simulink model "TESTS"  (R2022b)
settings: Solver=ode4  StartTime=0.0  StopTime=10.0  FixedStep=1e-4  RelTol=1e-3
values from neighbouring files (symbols this model uses):
  cel_serie = 6    [init_VE_EPRM_24_25.m]
  ke = 0.107    [init_VE_EPRM_24_25.m]
  ki = ke    (= 0.107)    [init_VE_EPRM_24_25.m]
  Kie = Kpe/taue    (= 9.6)    [init_VE_EPRM_24_25.m]
  Kpe = taue/(gaine*tftbe)    (= 0.045)    [init_VE_EPRM_24_25.m]
  Kpm = Mv/taum    (= 8850)    [init_VE_EPRM_24_25.m]
  kred = 75/22    (= 3.40909090909)    [init_VE_EPRM_24_25.m]
  Lmcc = vbat/(2*fdec*Deltai)    (= 0.00015)    [init_VE_EPRM_24_25.m]
  mod_serie = 4    [init_VE_EPRM_24_25.m]
  Mv = 295    [init_VE_EPRM_24_25.m]
  n = 0.92    [init_VE_EPRM_24_25.m]
  r = (279.4*10^-3)/2    (= 0.1397)    [init_VE_EPRM_24_25.m]
  Rcell = 0.53*10^-3    (= 0.00053)    [init_VE_EPRM_24_25.m]
  Rmcc = 0.032    [init_VE_EPRM_24_25.m]
  Voc = 2    [init_VE_EPRM_24_25.m]
libraries: slpidlib x1, simulink x1
settings Model: Creator=ZinouAb  LastModifiedBy=ZinouAb

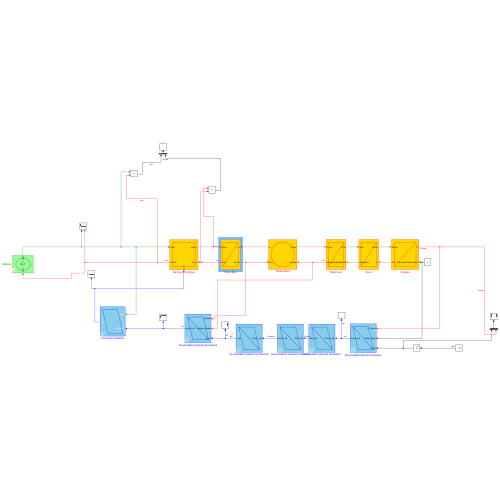
[thumbnail: Simulink's stored preview of the top-level diagram]
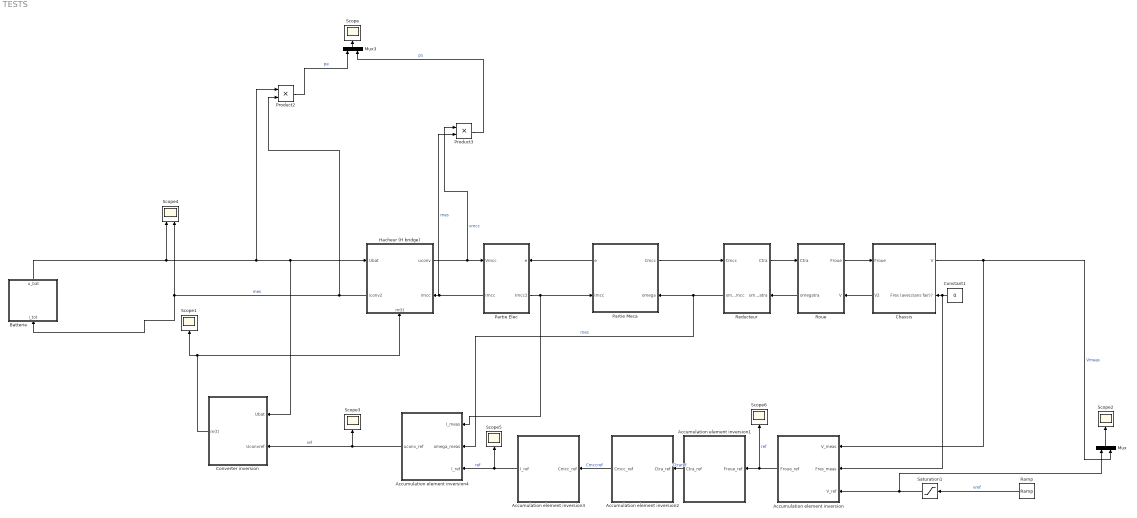
== system TESTS ==
  Accumulation element inversion : Subsystem  AncestorBlock=simulink/SMC/Asservissement Correcteur IP
      settings: LibrarySourceBlock=|
      | simulink/SMC/Asservissement
      | Correcteur IP
      mask Display: plot(0,0,100,100, [10,30,90,70,10,90],[90,10,10,90,90,10])
  Accumulation element inversion1 : Subsystem  AncestorBlock=simulink/SMC/Asservissement Correcteur IP
      settings: LibrarySourceBlock=|
      | simulink/SMC/Asservissement
      | Correcteur IP
      mask Display: plot(0,0,100,100, [10,30,90,70,10,90],[90,10,10,90,90,10])
  Accumulation element inversion2 : Subsystem  AncestorBlock=simulink/SMC/Asservissement Correcteur IP
      settings: LibrarySourceBlock=|
      | simulink/SMC/Asservissement
      | Correcteur IP
      mask Display: plot(0,0,100,100, [10,30,90,70,10,90],[90,10,10,90,90,10])
  Accumulation element inversion3 : Subsystem  AncestorBlock=simulink/SMC/Asservissement Correcteur IP
      settings: LibrarySourceBlock=|
      | simulink/SMC/Asservissement
      | Correcteur IP
      mask Display: plot(0,0,100,100, [10,30,90,70,10,90],[90,10,10,90,90,10])
  Accumulation element inversion4 : Subsystem  AncestorBlock=simulink/SMC/Asservissement Correcteur IP
      settings: LibrarySourceBlock=|
      | simulink/SMC/Asservissement
      | Correcteur IP
      mask Display: plot(0,0,100,100, [10,30,90,70,10,90],[90,10,10,90,90,10])
  Batterie : Subsystem  AncestorBlock=simulink/REM/SE
      settings: LibrarySourceBlock=simulink/REM/SE
      mask Display:
      | plot(0,0,100,100, 1.2*[50,57.68,60.77,63.08,64.97,66.58,68,69.26,70.4, 	71.42,72.36,78.28,80,78.28,72.36,71.42,70.4, 	69.26,68,66.58,64.97,63.08,60.77,57.68,50,42.32, 	39.23,36.92,35.03,33.42,32,30.74,29.6,28.58, 	27.64,21.72,20,21.72,27.64,28.58,29.6,30.74,32, 	33.42,35.03,36.92,39.23,42.32,50]-10, 1.2*[20,21,22,23,24,25,26,27,28,29,30,40,50,60,70,71,72, 	73,74,75,76,77,78,79,80,79,78,77,76,75,74,73,72, 	71,70,60,50,40,30,29,28,27,26,25,24,23,22,21,20]-10)
      | disp('BAT')
  Chassis : Subsystem
      settings: PortSchema="{\"entries\":[{\"content\":{\"sides\":[{\"content\":{\"connectorIds\":[\"In1\",\"Out2\"]},\"type\":\"ConnectorPlacement.EquallySpacedRectSide\",\"uuid\":\"2a4fefbc-7af2-45ac-94e1-720f9d1a181b\"},{\"content\":{\"connectorIds\":[\"Out1\",\"In2\"],\"side\":\"RIGHT\"},\"type\":\"ConnectorPlacement.EquallySpacedRectSide\",\"uuid\":\"47213f8a-38f1-43b2-8885-5842ee71090a\"},{\"content\":{\"connectorIds\":[],\"side\":\"TOP\"},\"type\":\"ConnectorPlacement.EquallySpacedRectSide\",\"uuid\":\"9ff55915-a798-409c-870e-d15a860382f9\"}]},\"type\":\"ConnectorPlacement.EquallySpacedConnector\",\"uuid\":\"647a32d4-94be-4190-bdc8-90a1a32d4cbf\"}],\"packageUris\":[\"http://schema.mathworks.com/mf0/Connector/R2020b\"],\"version\":\"1.0\"}"
      mask Display: plot(0,0,100,100,[10,10,90,90,10],[90,10,10,90,90], [10,90],[10,90])
  Constant1 : Constant  Value=0
  Converter inversion : Subsystem  AncestorBlock=simulink/SMC/Inversion EC avec mesure
      settings: LibrarySourceBlock=|
      | simulink/SMC/Inversion EC
      | avec mesure
      mask Display: plot(0,0,100,100,[10,30,90,70,10],[90,10,10,90,90])
  Hacheur (H bridge) : Subsystem
      settings: PortSchema="{\"entries\":[{\"content\":{\"sides\":[{\"content\":{\"connectorIds\":[\"In1\",\"Out2\"]},\"type\":\"ConnectorPlacement.EquallySpacedRectSide\",\"uuid\":\"15c37a82-4fae-4dd0-ab5a-78fb718c05e2\"},{\"content\":{\"connectorIds\":[\"Out1\",\"In3\"],\"side\":\"RIGHT\"},\"type\":\"ConnectorPlacement.EquallySpacedRectSide\",\"uuid\":\"2898708c-5198-4fba-9c94-abd5bb9e9c70\"},{\"content\":{\"connectorIds\":[],\"side\":\"TOP\"},\"type\":\"ConnectorPlacement.EquallySpacedRectSide\",\"uuid\":\"a769b592-c34b-45c3-8b04-17631095b399\"},{\"content\":{\"connectorIds\":[\"In2\"],\"side\":\"BOTTOM\"},\"type\":\"ConnectorPlacement.EquallySpacedRectSide\",\"uuid\":\"3f87bc4b-31a4-497c-9119-c9de1168f7cf\"}]},\"type\":\"ConnectorPlacement.EquallySpacedConnector\",\"uuid\":\"cf4da0bd-1e1f-410f-93a1-c54772eba95e\"}],\"packageUris\":[\"http://schema.mathworks.com/mf0/Connector/R2020b\"],\"version\":\"1.0\"}"
      mask Display: plot(0,0,100,100,[10,10,90,90,10],[90,10,10,90,90])
  Mux : Mux  Inputs=2
  Mux3 : Mux  Inputs=2
  Partie Elec : Subsystem
      settings: PortSchema="{\"entries\":[{\"content\":{\"sides\":[{\"content\":{\"connectorIds\":[\"In1\",\"Out2\"]},\"type\":\"ConnectorPlacement.EquallySpacedRectSide\",\"uuid\":\"2a4fefbc-7af2-45ac-94e1-720f9d1a181b\"},{\"content\":{\"connectorIds\":[\"In2\",\"Out1\"],\"side\":\"RIGHT\"},\"type\":\"ConnectorPlacement.EquallySpacedRectSide\",\"uuid\":\"47213f8a-38f1-43b2-8885-5842ee71090a\"},{\"content\":{\"connectorIds\":[],\"side\":\"TOP\"},\"type\":\"ConnectorPlacement.EquallySpacedRectSide\",\"uuid\":\"9ff55915-a798-409c-870e-d15a860382f9\"}]},\"type\":\"ConnectorPlacement.EquallySpacedConnector\",\"uuid\":\"647a32d4-94be-4190-bdc8-90a1a32d4cbf\"}],\"packageUris\":[\"http://schema.mathworks.com/mf0/Connector/R2020b\"],\"version\":\"1.0\"}"
      mask Display: plot(0,0,100,100,[10,10,90,90,10],[90,10,10,90,90], [10,90],[10,90])
  Partie Meca : Subsystem
      settings: PortSchema="{\"entries\":[{\"content\":{\"sides\":[{\"content\":{\"connectorIds\":[\"Out2\",\"In1\"]},\"type\":\"ConnectorPlacement.EquallySpacedRectSide\",\"uuid\":\"2a4fefbc-7af2-45ac-94e1-720f9d1a181b\"},{\"content\":{\"connectorIds\":[\"Out1\",\"In2\"],\"side\":\"RIGHT\"},\"type\":\"ConnectorPlacement.EquallySpacedRectSide\",\"uuid\":\"47213f8a-38f1-43b2-8885-5842ee71090a\"},{\"content\":{\"connectorIds\":[],\"side\":\"TOP\"},\"type\":\"ConnectorPlacement.EquallySpacedRectSide\",\"uuid\":\"9ff55915-a798-409c-870e-d15a860382f9\"}]},\"type\":\"ConnectorPlacement.EquallySpacedConnector\",\"uuid\":\"647a32d4-94be-4190-bdc8-90a1a32d4cbf\"}],\"packageUris\":[\"http://schema.mathworks.com/mf0/Connector/R2020b\"],\"version\":\"1.0\"}"
      mask Display: plot(0,0,100,100, 1.4*[50,57.68,60.77,63.08,64.97,66.58,68,69.26,70.4, 	71.42,72.36,78.28,80,78.28,72.36,71.42,70.4, 	69.26,68,66.58,64.97,63.08,60.77,57.68,50,42.32, 	39.23,36.92,35.03,33.42,32,30.74,29.6,28.58, 	27.64,21.72,20,21.72,27.64,28.58,29.6,30.74,32, 	33.42,35.03,36.92,39.23,42.32,50]-20, 1.4*[20,21,22,23,24,25,26,27,28,29,30,40,50,60,70,71,72, 	73,74,75,76,77,78,79,80,79,78,77,76,75,74,73,72, 	71,70,60,50,40,30,29,28,27,26,25,24,23,22,21,20]-20)
  Product2 : Product
  Product3 : Product
  Ramp : simulink/Sources/Ramp  slope=1  start=1  InitialOutput=0
  Reducteur : Subsystem
      settings: PortSchema="{\"entries\":[{\"content\":{\"sides\":[{\"content\":{\"connectorIds\":[\"In1\",\"Out2\"]},\"type\":\"ConnectorPlacement.EquallySpacedRectSide\",\"uuid\":\"2a4fefbc-7af2-45ac-94e1-720f9d1a181b\"},{\"content\":{\"connectorIds\":[\"Out1\",\"In2\"],\"side\":\"RIGHT\"},\"type\":\"ConnectorPlacement.EquallySpacedRectSide\",\"uuid\":\"47213f8a-38f1-43b2-8885-5842ee71090a\"},{\"content\":{\"connectorIds\":[],\"side\":\"TOP\"},\"type\":\"ConnectorPlacement.EquallySpacedRectSide\",\"uuid\":\"9ff55915-a798-409c-870e-d15a860382f9\"}]},\"type\":\"ConnectorPlacement.EquallySpacedConnector\",\"uuid\":\"647a32d4-94be-4190-bdc8-90a1a32d4cbf\"}],\"packageUris\":[\"http://schema.mathworks.com/mf0/Connector/R2020b\"],\"version\":\"1.0\"}"
      mask Display: plot(0,0,100,100,[10,10,90,90,10],[90,10,10,90,90], [10,90],[10,90])
  Roue : Subsystem
      settings: PortSchema="{\"entries\":[{\"content\":{\"sides\":[{\"content\":{\"connectorIds\":[\"In1\",\"Out2\"]},\"type\":\"ConnectorPlacement.EquallySpacedRectSide\",\"uuid\":\"2a4fefbc-7af2-45ac-94e1-720f9d1a181b\"},{\"content\":{\"connectorIds\":[\"Out1\",\"In2\"],\"side\":\"RIGHT\"},\"type\":\"ConnectorPlacement.EquallySpacedRectSide\",\"uuid\":\"47213f8a-38f1-43b2-8885-5842ee71090a\"},{\"content\":{\"connectorIds\":[],\"side\":\"TOP\"},\"type\":\"ConnectorPlacement.EquallySpacedRectSide\",\"uuid\":\"9ff55915-a798-409c-870e-d15a860382f9\"}]},\"type\":\"ConnectorPlacement.EquallySpacedConnector\",\"uuid\":\"647a32d4-94be-4190-bdc8-90a1a32d4cbf\"}],\"packageUris\":[\"http://schema.mathworks.com/mf0/Connector/R2020b\"],\"version\":\"1.0\"}"
      mask Display: plot(0,0,100,100,[10,10,90,90,10],[90,10,10,90,90], [10,90],[10,90])
  Saturation1 : Saturate  UpperLimit=1  LowerLimit=-1  LinearizeAsGain=off
  Scope{,1..3,5..6} (6 alike) : Scope
  Scope4 : Scope  NumInputPorts=2
  wires:
  Accumulation element inversion4/1(uconv_ref) -> Scope3/1, Converter inversion/2("Uconvref ")  "ref"
  Converter inversion/1(m(t)) -> Hacheur (H bridge)/2(m(t)), Scope1/1
  Partie Elec/1(Imcc2) -> Partie Meca/1(Imcc), Accumulation element inversion4/1(I_meas)
  Product3/1 -> Mux3/2  "ps"
  Mux3/1 -> Scope/1
  Product2/1 -> Mux3/1  "pe"
  Hacheur (H bridge)/1("uconv ") -> Product3/1, Partie Elec/1(Vmcc)  "vmcc"
  Mux/1 -> Scope2/1
  Partie Meca/2(e) -> Partie Elec/2(e)
  Reducteur/1(Ctra) -> Roue/1(Ctra)
  Roue/2(omegatra) -> Reducteur/2(omegatra)
  Roue/1(Froue) -> Chassis/1(Froue)
  Chassis/2(V2) -> Roue/2(V)
  Partie Meca/1(Cmcc) -> Reducteur/1(Cmcc)
  Reducteur/2(omegamcc) -> Accumulation element inversion4/2(omega_meas), Partie Meca/2(omega)  "mes"
  Constant1/1 -> Accumulation element inversion/2(Fres_meas), Chassis/2(Fres (avec/sans fair)?)
  Chassis/1(V) -> Mux/2, Accumulation element inversion/1(V_meas)  "Vmeas"
  Accumulation element inversion1/1(Ctra_ref) -> Accumulation element inversion2/1(Ctra_ref)  "Ctraref"
  Accumulation element inversion2/1(Cmcc_ref) -> Accumulation element inversion3/1(Cmcc_ref)  "Cmccref"
  Hacheur (H bridge)/2(iconv2) -> Product2/2, Batterie/1(i_tot), Scope4/2  "mes"
  Batterie/1(u_bat) -> Scope4/1, Product2/1, Converter inversion/1(Ubat), Hacheur (H bridge)/1("Ubat ")
  Partie Elec/2(Imcc) -> Hacheur (H bridge)/3("imcc "), Product3/2  "mes"
  Accumulation element inversion3/1(I_ref) -> Scope5/1, Accumulation element inversion4/3(I_ref)  "ref"
  Accumulation element inversion/1(Froue_ref) -> Scope6/1, Accumulation element inversion1/1(Froue_ref)  "ref"
  Saturation1/1 -> Mux/1, Accumulation element inversion/3(V_ref)
  Ramp/1 -> Saturation1/1  "vref"

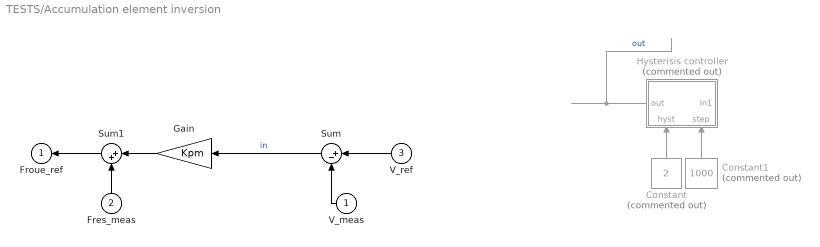
== system TESTS/Accumulation element inversion ==
  V_meas : Inport
  Fres_meas : Inport  Port=2
  V_ref : Inport  Port=3
  Constant : Constant  Commented=on  Value=2
  Constant1 : Constant  Commented=on  Value=1000
  Gain : Gain  Gain=Kpm
  Hysterisis controller : Subsystem  Commented=on
      settings: PortSchema="{\"entries\":[{\"content\":{\"sides\":[{\"content\":{\"connectorIds\":[\"In1\"]},\"type\":\"ConnectorPlacement.EquallySpacedRectSide\",\"uuid\":\"f66aa083-2ee8-4426-b441-0f8ce3c91bc6\"},{\"content\":{\"connectorIds\":[\"Out1\"],\"side\":\"RIGHT\"},\"type\":\"ConnectorPlacement.EquallySpacedRectSide\",\"uuid\":\"e535ff9d-11f2-429a-8d26-bff265e6dce4\"},{\"content\":{\"connectorIds\":[\"In2\",\"In3\"],\"side\":\"TOP\"},\"type\":\"ConnectorPlacement.EquallySpacedRectSide\",\"uuid\":\"3bf3f486-5ffc-4655-8aef-50265858aab1\"},{\"content\":{\"connectorIds\":[],\"side\":\"BOTTOM\"},\"type\":\"ConnectorPlacement.EquallySpacedRectSide\",\"uuid\":\"619b2421-7bbc-4c41-b693-a17d0c478cc9\"}]},\"type\":\"ConnectorPlacement.EquallySpacedConnector\",\"uuid\":\"4c23f3cf-154a-4c58-b671-46cc18db332d\"}],\"packageUris\":[\"http://schema.mathworks.com/mf0/Connector/R2020b\"],\"version\":\"1.0\"}"
  Sum : Sum  Inputs=|+-
  Sum1 : Sum  Inputs=|++
  Froue_ref : Outport  InitialOutput=0
  wires:
  Hysterisis controller/1(out) -> ?  "out"
  Sum/1 -> Gain/1  "in"
  Constant/1 -> Hysterisis controller/3(hyst)
  Fres_meas/1 -> Sum1/2
  Sum1/1 -> Froue_ref/1
  ? -> Hysterisis controller/1(In1)  "in"
  Constant1/1 -> Hysterisis controller/2(step)
  V_ref/1 -> Sum/1
  V_meas/1 -> Sum/2
  Gain/1 -> Sum1/1

== system TESTS/Accumulation element inversion1 ==
  Froue_ref : Inport
  Gain : Gain  Gain=r
  Ctra_ref : Outport  InitialOutput=0
  wires:
  Gain/1 -> Ctra_ref/1
  Froue_ref/1 -> Gain/1

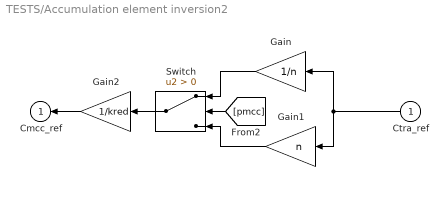
== system TESTS/Accumulation element inversion2 ==
  Ctra_ref : Inport
  Gain : Gain  Gain=1/n
  Gain1 : Gain  Gain=n
  Gain2 : Gain  Gain=1/kred
  Switch : Switch  Criteria=u2 > Threshold  SaturateOnIntegerOverflow=off  InputSameDT=off
  Cmcc_ref : Outport  InitialOutput=0
  wires:
  Switch/1 -> Gain2/1
  Ctra_ref/1 -> Gain/1, Gain1/1
  [pmcc] -> Switch/2
  Gain/1 -> Switch/1
  Gain1/1 -> Switch/3
  Gain2/1 -> Cmcc_ref/1

== system TESTS/Accumulation element inversion3 ==
  Cmcc_ref : Inport
  Gain : Gain  Gain=1/ki
  I_ref : Outport  InitialOutput=0
  wires:
  Gain/1 -> I_ref/1
  Cmcc_ref/1 -> Gain/1

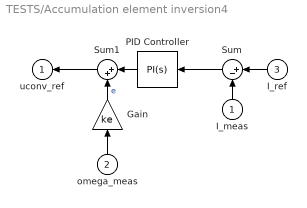
== system TESTS/Accumulation element inversion4 ==
  I_meas : Inport
  omega_meas : Inport  Port=2
  I_ref : Inport  Port=3
  Gain : Gain  Gain=ke
  PID Controller : slpidlib/PID Controller  Controller=PI  Form=Parallel  TimeDomain=Continuous-time  UseExternalTs=off  SampleTime=-1  IntegratorMethod=Forward Euler  FilterMethod=Forward Euler  ControllerParametersSource=internal  P=Kpe  I=Kie  UseKiTs=off  D=0  N=100  UseFilter=on  TunerSelectOption=Transfer Function Based (PID Tuner App)  InitialConditionSource=internal  InitialConditionForIntegrator=0  InitialConditionForFilter=0  DifferentiatorICPrevScaledInput=0  ExternalReset=none  TrackingMode=off  Kt=1  LimitOutput=off  SatLimitsSource=internal  UpperSaturationLimit=inf  LowerSaturationLimit=-inf  LinearizeAsGain=on  AntiWindupMode=none  Kb=1  LimitIntegrator=off  UpperIntegratorSaturationLimit=inf  LowerIntegratorSaturationLimit=-inf  POutMin=[]  POutMax=[]  IOutMin=[]  IOutMax=[]  DOutMin=[]  DOutMax=[]  NOutMin=[]  NOutMax=[]  SumOutMin=[]  SumOutMax=[]  SaturationOutMin=[]  SaturationOutMax=[]  PParamMin=[]  PParamMax=[]  IParamMin=[]  IParamMax=[]  DParamMin=[]  DParamMax=[]  NParamMin=[]  NParamMax=[]  KbParamMin=[]  KbParamMax=[]  KtParamMin=[]  KtParamMax=[]  KbOutMin=[]  KbOutMax=[]  KtOutMin=[]  KtOutMax=[]  IntegratorOutMin=[]  IntegratorOutMax=[]  FilterOutMin=[]  FilterOutMax=[]  SumI1OutMin=[]  SumI1OutMax=[]  SumI2OutMin=[]  SumI2OutMax=[]  SumI3OutMin=[]  SumI3OutMax=[]  SumI4OutMin=[]  SumI4OutMax=[]  SumDOutMin=[]  SumDOutMax=[]  DifferentiatorOutMin=[]  DifferentiatorOutMax=[]  FilterDiffOutCoefMin=[]  FilterDiffOutCoefMax=[]  ReciprocalOutMin=[]  ReciprocalOutMax=[]  SumDenOutMin=[]  SumDenOutMax=[]  SumNumOutMin=[]  SumNumOutMax=[]  DivideOutMin=[]  DivideOutMax=[]  UdiffTsProdOutMin=[]  UdiffTsProdOutMax=[]  NTsProdOutMin=[]  NTsProdOutMax=[]  UintegralTsProdOutMin=[]  UintegralTsProdOutMax=[]  UngainTsProdOutMin=[]  UngainTsProdOutMax=[]  ClampingZeroOutDataTypeStr=Inherit: Inherit via back propagation  ClampingZeroOutMin=[]  ClampingZeroOutMax=[]  FilterDenConstantOutDataTypeStr=Inherit: Inherit via back propagation  FilterDenConstantOutMin=[]  FilterDenConstantOutMax=[]  PCopyOutDataTypeStr=Inherit: Inherit via back propagation  PCopyOutMin=[]  PCopyOutMax=[]  NCopyOutDataTypeStr=Inherit: Inherit via back propagation  NCopyOutMin=[]  NCopyOutMax=[]  IntegratorContinuousStateAttributes=''  IntegratorStateMustResolveToSignalObject=off  IntegratorRTWStateStorageClass=Auto  FilterContinuousStateAttributes=''  FilterStateMustResolveToSignalObject=off  FilterRTWStateStorageClass=Auto  ParallelPVariant=InternalParameters  IdealPVariant=Disabled  IVariant=InternalParameters  DVariant=Disabled  IntegratorVariant=Continuous  SatVariant=Disabled  AWVariant=Passthrough  PCopyVariant=Disabled  TRVariant=Disabled  FdbkBlocksVariant=Forward  IdealPFdbkVariant=Disabled  SatFdbkVariant=Disabled  DerivativeFilterVariant=Disabled  NVariant=Disabled  NCopyVariant=Disabled_SignalSpec  FilterICVariant=Disabled  IntegratorICVariant=InternalICs  ExternalResetVariant=Disabled  TRSumVariant=Passthrough  SumFdbkVariant=Disabled  SumVariant=Sum_PI  TsampFilterVariant=InternalTs  TsampNgainVariant=Passthrough  TsampIntegralVariant=Passthrough  ExternalSaturationOutDataTypeStr=Inherit: Same as second input
  Sum : Sum  Inputs=|+-
  Sum1 : Sum  Inputs=|++
  uconv_ref : Outport  InitialOutput=0
  wires:
  I_meas/1 -> Sum/2
  omega_meas/1 -> Gain/1
  Sum/1 -> PID Controller/1
  Sum1/1 -> uconv_ref/1
  Gain/1 -> Sum1/2  "e"
  PID Controller/1 -> Sum1/1
  I_ref/1 -> Sum/1

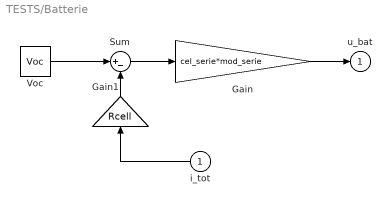
== system TESTS/Batterie ==
  i_tot : Inport
  Gain : Gain  Gain=cel_serie*mod_serie
  Gain1 : Gain  Gain=Rcell
  Sum : Sum  Inputs=|+-
  Voc : Constant  Value=Voc
  u_bat : Outport  InitialOutput=0
  wires:
  Voc/1 -> Sum/1
  Sum/1 -> Gain/1
  Gain1/1 -> Sum/2
  Gain/1 -> u_bat/1
  i_tot/1 -> Gain1/1

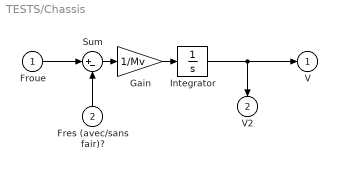
== system TESTS/Chassis ==
  Froue : Inport
  Fres (avec/sans fair)? : Inport  Port=2
  Gain : Gain  Gain=1/Mv
  Integrator : Integrator
  Sum : Sum  Inputs=|+-
  V : Outport  InitialOutput=0
  V2 : Outport  Port=2  InitialOutput=0
  wires:
  Integrator/1 -> V2/1, V/1
  Froue/1 -> Sum/1
  Sum/1 -> Gain/1
  Gain/1 -> Integrator/1
  Fres (avec/sans fair)?/1 -> Sum/2

== system TESTS/Converter inversion ==
  Ubat : Inport
  "Uconvref " : Inport  Port=2
  Divide : Product  Inputs=*/
  Memory : Memory  InitialCondition=48
  m(t) : Outport  InitialOutput=0
  wires:
  Ubat/1 -> Memory/1
  Divide/1 -> m(t)/1
  "Uconvref "/1 -> Divide/1
  Memory/1 -> Divide/2

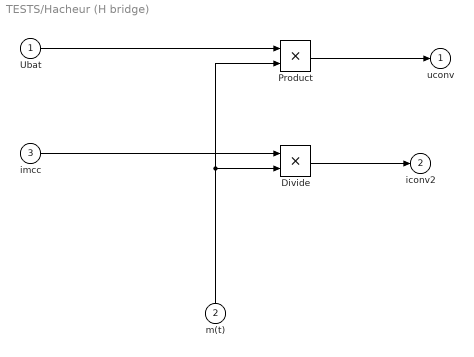
== system TESTS/Hacheur (H bridge) ==
  "Ubat " : Inport
  m(t) : Inport  Port=2
  "imcc " : Inport  Port=3
  Divide : Product  Inputs=**
  Product : Product
  "uconv " : Outport  InitialOutput=0
  iconv2 : Outport  Port=2  InitialOutput=0
  wires:
  m(t)/1 -> Divide/2, Product/2
  "Ubat "/1 -> Product/1
  "imcc "/1 -> Divide/1
  Divide/1 -> iconv2/1
  Product/1 -> "uconv "/1

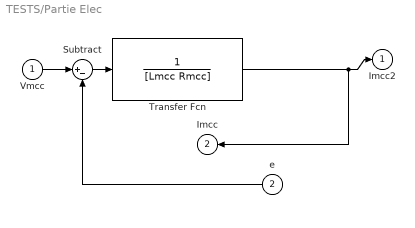
== system TESTS/Partie Elec ==
  Vmcc : Inport
  e : Inport  Port=2
  Subtract : Sum  Inputs=|+-
  Transfer Fcn : TransferFcn  Denominator=[Lmcc Rmcc]
  Imcc2 : Outport  InitialOutput=0
  Imcc : Outport  Port=2  InitialOutput=0
  wires:
  e/1 -> Subtract/2
  Subtract/1 -> Transfer Fcn/1
  Vmcc/1 -> Subtract/1
  Transfer Fcn/1 -> Imcc/1, Imcc2/1

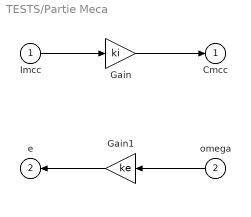
== system TESTS/Partie Meca ==
  Imcc : Inport
  omega : Inport  Port=2
  Gain : Gain  Gain=ki
  Gain1 : Gain  Gain=ke
  Cmcc : Outport  InitialOutput=0
  e : Outport  Port=2  InitialOutput=0
  wires:
  omega/1 -> Gain1/1
  Imcc/1 -> Gain/1
  Gain1/1 -> e/1
  Gain/1 -> Cmcc/1

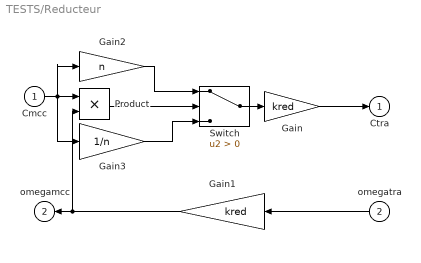
== system TESTS/Reducteur ==
  Cmcc : Inport
  omegatra : Inport  Port=2
  Gain : Gain  Gain=kred
  Gain1 : Gain  Gain=kred
  Gain2 : Gain  Gain=n
  Gain3 : Gain  Gain=1/n
  Product : Product
  Switch : Switch  Criteria=u2 > Threshold  SaturateOnIntegerOverflow=off  InputSameDT=off
  Ctra : Outport  InitialOutput=0
  omegamcc : Outport  Port=2  InitialOutput=0
  wires:
  omegatra/1 -> Gain1/1
  Gain1/1 -> Product/2, omegamcc/1
  Cmcc/1 -> Gain3/1, Gain2/1, Product/1
  Gain/1 -> Ctra/1
  Product/1 -> Switch/2
  Switch/1 -> Gain/1
  Gain3/1 -> Switch/3
  Gain2/1 -> Switch/1

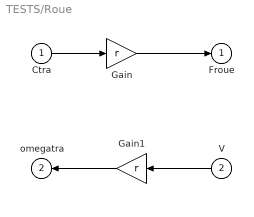
== system TESTS/Roue ==
  Ctra : Inport
  V : Inport  Port=2
  Gain : Gain  Gain=r
  Gain1 : Gain  Gain=r
  Froue : Outport  InitialOutput=0
  omegatra : Outport  Port=2  InitialOutput=0
  wires:
  V/1 -> Gain1/1
  Ctra/1 -> Gain/1
  Gain1/1 -> omegatra/1
  Gain/1 -> Froue/1

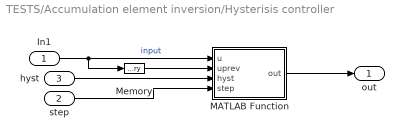
== system TESTS/Accumulation element inversion/Hysterisis controller ==
  In1 : Inport
  step : Inport  Port=2
  hyst : Inport  Port=3
  MATLAB Function : MATLAB Function  TreatAsAtomicUnit=on
  Memory : Memory
  out : Outport
  wires:
  In1/1 -> Memory/1, MATLAB Function/1(u)  "input"
  Memory/1 -> MATLAB Function/2(uprev)
  MATLAB Function/1(out) -> out/1
  step/1 -> MATLAB Function/4(step)
  hyst/1 -> MATLAB Function/3(hyst)

== matlab function TESTS/Accumulation element inversion/Hysterisis controller/MATLAB Function ==
  data: u input; out output; uprev input; hyst input; step input
function out = hystcontrol(u,uprev,hyst,step)

if u>hyst
    out= uprev-step;
elseif u<hyst
    out= uprev+step;
else
    out=uprev;

end
